simulink model "SF009A_DutyCycThermProtn"  (R2013b)
settings: Solver=FixedStepDiscrete  SolverMode=SingleTasking  StartTime=0.0  StopTime=1  FixedStep=0.1  RelTol=1e-3
values from neighbouring files (symbols this model uses):
  AbsltTThermLimCnt = DataDict.NTC    [SF009A_DutyCycThermProtn_DataDict.m]
  ARCHGLBPRM_100MILLISEC_SEC_F32 = DataDict.Constant    [SF009A_DutyCycThermProtn_DataDict.m]
  CTRLRANDCUTFLT_CNT_U08 = DataDict.Constant    [SF009A_DutyCycThermProtn_DataDict.m]
  CTRLRTFLT_CNT_U08 = DataDict.Constant    [SF009A_DutyCycThermProtn_DataDict.m]
  CUTFLT_CNT_U08 = DataDict.Constant    [SF009A_DutyCycThermProtn_DataDict.m]
  DITHERMLIM_MOTNWTMTR_F32 = DataDict.Constant    [SF009A_DutyCycThermProtn_DataDict.m]
  DutyCycExcddCnt = DataDict.NTC    [SF009A_DutyCycThermProtn_DataDict.m]
  DutyCycThermProtnAbsltCtrlTTblX = DataDict.Calibration    [SF009A_DutyCycThermProtn_DataDict.m]
  DutyCycThermProtnAbsltCtrlTTqTblY = DataDict.Calibration    [SF009A_DutyCycThermProtn_DataDict.m]
  DutyCycThermProtnAbsltCuTTblX = DataDict.Calibration    [SF009A_DutyCycThermProtn_DataDict.m]
  DutyCycThermProtnAbsltCuTTqTblY = DataDict.Calibration    [SF009A_DutyCycThermProtn_DataDict.m]
  DutyCycThermProtnAbsltMotVelBreakPt = DataDict.Calibration    [SF009A_DutyCycThermProtn_DataDict.m]
  DutyCycThermProtnAbsltTTqSlewHiLim = DataDict.Calibration    [SF009A_DutyCycThermProtn_DataDict.m]
  DutyCycThermProtnAbsltTTqSlewLoLim = DataDict.Calibration    [SF009A_DutyCycThermProtn_DataDict.m]
  DutyCycThermProtnCtrlT = DataDict.Calibration    [SF009A_DutyCycThermProtn_DataDict.m]
  DutyCycThermProtnCtrlTSeln = DataDict.Calibration    [SF009A_DutyCycThermProtn_DataDict.m]
  DutyCycThermProtnDutyCycFildThd = DataDict.Calibration    [SF009A_DutyCycThermProtn_DataDict.m]
  DutyCycThermProtnIgnOffCtrlEna = DataDict.Calibration    [SF009A_DutyCycThermProtn_DataDict.m]
  DutyCycThermProtnIgnOffMsgWaitTi = DataDict.Calibration    [SF009A_DutyCycThermProtn_DataDict.m]
  DutyCycThermProtnLstTblValNonStall = DataDict.Calibration    [SF009A_DutyCycThermProtn_DataDict.m]
  DutyCycThermProtnLstTblValStall = DataDict.Calibration    [SF009A_DutyCycThermProtn_DataDict.m]
  DutyCycThermProtnMotPrTSeln = DataDict.Calibration    [SF009A_DutyCycThermProtn_DataDict.m]
  DutyCycThermProtnMplr1NonStallTblY = DataDict.Calibration    [SF009A_DutyCycThermProtn_DataDict.m]
  DutyCycThermProtnMplr1StallTblY = DataDict.Calibration    [SF009A_DutyCycThermProtn_DataDict.m]
  DutyCycThermProtnMplr2NonStallTblY = DataDict.Calibration    [SF009A_DutyCycThermProtn_DataDict.m]
  DutyCycThermProtnMplr2StallTblY = DataDict.Calibration    [SF009A_DutyCycThermProtn_DataDict.m]
  DutyCycThermProtnMplr3NonStallTblY = DataDict.Calibration    [SF009A_DutyCycThermProtn_DataDict.m]
  DutyCycThermProtnMplr3StallTblY = DataDict.Calibration    [SF009A_DutyCycThermProtn_DataDict.m]
  DutyCycThermProtnMplr4NonStallTblY = DataDict.Calibration    [SF009A_DutyCycThermProtn_DataDict.m]
  DutyCycThermProtnMplr4StallTblY = DataDict.Calibration    [SF009A_DutyCycThermProtn_DataDict.m]
  DutyCycThermProtnMplr5NonStallTblY = DataDict.Calibration    [SF009A_DutyCycThermProtn_DataDict.m]
  DutyCycThermProtnMplr5StallTblY = DataDict.Calibration    [SF009A_DutyCycThermProtn_DataDict.m]
  DutyCycThermProtnMplr6NonStallTblY = DataDict.Calibration    [SF009A_DutyCycThermProtn_DataDict.m]
  DutyCycThermProtnMplr6StallTblY = DataDict.Calibration    [SF009A_DutyCycThermProtn_DataDict.m]
  DutyCycThermProtnMplrTblX = DataDict.Calibration    [SF009A_DutyCycThermProtn_DataDict.m]
  DutyCycThermProtnMplrTSeln = DataDict.Calibration    [SF009A_DutyCycThermProtn_DataDict.m]
  DutyCycThermProtnSlowFilTSeln = DataDict.Calibration    [SF009A_DutyCycThermProtn_DataDict.m]
  DutyCycThermProtnThermLimScaFac = DataDict.Calibration    [SF009A_DutyCycThermProtn_DataDict.m]
  DutyCycThermProtnThermLoadLimTblX = DataDict.Calibration    [SF009A_DutyCycThermProtn_DataDict.m]
  DutyCycThermProtnThermLoadLimTblY = DataDict.Calibration    [SF009A_DutyCycThermProtn_DataDict.m]
  DutyCycThermProtnTqCmdSlewDwn = DataDict.Calibration    [SF009A_DutyCycThermProtn_DataDict.m]
  DutyCycThermProtnTqCmdSlewUp = DataDict.Calibration    [SF009A_DutyCycThermProtn_DataDict.m]
  FILVALMIN_ULS_F32 = DataDict.Constant    [SF009A_DutyCycThermProtn_DataDict.m]
  IGNTIOFFTHD_CNT_F32 = DataDict.Constant    [SF009A_DutyCycThermProtn_DataDict.m]
  NODEBSTEP_CNT_U16 = DataDict.Constant    [SF009A_DutyCycThermProtn_DataDict.m]
  ONEPERC_ULS_F32 = DataDict.Constant    [SF009A_DutyCycThermProtn_DataDict.m]
  TAU3_SEC_F32 = DataDict.Constant    [SF009A_DutyCycThermProtn_DataDict.m]
  TAU4_SEC_F32 = DataDict.Constant    [SF009A_DutyCycThermProtn_DataDict.m]
  TAU5_SEC_F32 = DataDict.Constant    [SF009A_DutyCycThermProtn_DataDict.m]
  TAU6_SEC_F32 = DataDict.Constant    [SF009A_DutyCycThermProtn_DataDict.m]
  THERMLOADLIMTBLIDX_ULS_U08 = DataDict.Constant    [SF009A_DutyCycThermProtn_DataDict.m]
undefined symbols (not defined in the file or in its folder): NtcSts1, NvmGetErrSts1
libraries: FixdToFloat x13, Fil x12, NxtrLim x12, simulink x11, NxtrMath x8, FloatToFixd x6, NxtrMax x6, NxtrMin x3, NxtrAbslt x2, NxtrNvM x1
(part 5 of 7)

== system SF009A_DutyCycThermProtn/DutyCycThermProtn/DutyCycThermProtnPer1/TherrmalLimitScaling/ThermDutyCycLoadDptDisabled  ==
  Action Port : ActionPort  ActionType=then
  CopyRight2 : Subsystem  Description=|  mask(Copyright Information){none=on}
      | Copyright info block.                                               
      |                                                                     
      | Place copyright information at the top of every subsystem in design.
      mask prompts: none "No parameters"
      mask help: Place copyright information at the top of every subsystem in design.
      mask Display:
      | NxtrConf = 'Nexteer Confidential';
      | 
      | sys = bdroot; %handle for the current model ("system")
      | first = get_param(sys,'Created');
      | first = first(end-3:end);  %year is last four digits
      | 
      | last = get_param(sys,'LastModifiedDate');
      | if isempty(last)
      |     last = datestr(now,'yyyy');
      | else
      |     last = last(end-3:end);
      | end
      | 
      | if strcmp(first,last)
      |     fprintf('%s -- Copyright %s Nexteer',NxtrConf,first)
      | else
      |     fprintf('%s -- %s%s- %s Nexteer',NxtrConf,char(169),first,last)
      | end
  D_DEFEATTHERMLLIMIT_MTRNM : Constant  RequirementInfo="{'linktype_rmi_doors' '0000a52a (/E-STEER Core/SubSystem Specifications/Application Functions/SF009A Thermal Duty Cycle Protection)' '#SF009A_233' 'true' 'REQ:  SF009A_233' '' } %GIDa_fe9f7413_b640_416a_8163_cba554ef26c1"  Value=DITHERMLIM_MOTNWTMTR_F32
  ThermLdDptLim : Outport
  wires:
  D_DEFEATTHERMLLIMIT_MTRNM/1 -> ThermLdDptLim/1

== system SF009A_DutyCycThermProtn/DutyCycThermProtn/DutyCycThermProtnPer1/TherrmalLimitScaling/ThermDutyCycLoadDptEnabled ==
  ThermLoadDptLim : Inport
  Action Port : ActionPort  ActionType=else
  CopyRight2 : Subsystem  Description=|  mask(Copyright Information){none=on}
      | Copyright info block.                                               
      |                                                                     
      | Place copyright information at the top of every subsystem in design.
      mask prompts: none "No parameters"
      mask help: Place copyright information at the top of every subsystem in design.
      mask Display:
      | NxtrConf = 'Nexteer Confidential';
      | 
      | sys = bdroot; %handle for the current model ("system")
      | first = get_param(sys,'Created');
      | first = first(end-3:end);  %year is last four digits
      | 
      | last = get_param(sys,'LastModifiedDate');
      | if isempty(last)
      |     last = datestr(now,'yyyy');
      | else
      |     last = last(end-3:end);
      | end
      | 
      | if strcmp(first,last)
      |     fprintf('%s -- Copyright %s Nexteer',NxtrConf,first)
      | else
      |     fprintf('%s -- %s%s- %s Nexteer',NxtrConf,char(169),first,last)
      | end
  ThermLdDptLim : Outport
  wires:
  ThermLoadDptLim/1 -> ThermLdDptLim/1

== system SF009A_DutyCycThermProtn/DutyCycThermProtn/DutyCycThermProtnPer1/TherrmalLimitScaling/ThermLim_DutyCycThermProtnDisabled1 ==
  AbsTempLimitSlew : Inport
  Action Port : ActionPort  ActionType=then
  CopyRight2 : Subsystem  Description=|  mask(Copyright Information){none=on}
      | Copyright info block.                                               
      |                                                                     
      | Place copyright information at the top of every subsystem in design.
      mask prompts: none "No parameters"
      mask help: Place copyright information at the top of every subsystem in design.
      mask Display:
      | NxtrConf = 'Nexteer Confidential';
      | 
      | sys = bdroot; %handle for the current model ("system")
      | first = get_param(sys,'Created');
      | first = first(end-3:end);  %year is last four digits
      | 
      | last = get_param(sys,'LastModifiedDate');
      | if isempty(last)
      |     last = datestr(now,'yyyy');
      | else
      |     last = last(end-3:end);
      | end
      | 
      | if strcmp(first,last)
      |     fprintf('%s -- Copyright %s Nexteer',NxtrConf,first)
      | else
      |     fprintf('%s -- %s%s- %s Nexteer',NxtrConf,char(169),first,last)
      | end
  D_DEFEATTHERMLLIMIT_MTRNM : Constant  RequirementInfo="{'linktype_rmi_doors' '0000a52a (/E-STEER Core/SubSystem Specifications/Application Functions/SF009A Thermal Duty Cycle Protection)' '#SF009A_315' 'true' 'REQ:  SF009A_315' '' ; 'linktype_rmi_doors' '0000a52a (/E-STEER Core/SubSystem Specifications/Application Functions/SF009A Thermal Duty Cycle Protection)' '#SF009A_321' 'true' 'REQ:  SF009A_321' '' ; 'linktype_rmi_doors' '0000a52a (/E-STEER Core/SubSystem Specifications/Application Functions/SF009A Thermal Duty Cycle Protection)' '#SF009A_320' 'true' 'REQ:  SF009A_320' '' } %GIDa_b0686dc6_4c24_4aa9_95e9_6eecdcdad624"  Value=DutyCycThermProtnThermLimScaFac
  Product1 : Product  RndMeth=Zero
  ThermTempDptLmt : Outport
  wires:
  D_DEFEATTHERMLLIMIT_MTRNM/1 -> Product1/2
  Product1/1 -> ThermTempDptLmt/1
  AbsTempLimitSlew/1 -> Product1/1

== system SF009A_DutyCycThermProtn/DutyCycThermProtn/DutyCycThermProtnPer1/TherrmalLimitScaling/ThermLim_DutyCycThermProtnDisabled2 ==
  ThermalLoadLmt : Inport
  Action Port : ActionPort  ActionType=then
  CopyRight2 : Subsystem  Description=|  mask(Copyright Information){none=on}
      | Copyright info block.                                               
      |                                                                     
      | Place copyright information at the top of every subsystem in design.
      mask prompts: none "No parameters"
      mask help: Place copyright information at the top of every subsystem in design.
      mask Display:
      | NxtrConf = 'Nexteer Confidential';
      | 
      | sys = bdroot; %handle for the current model ("system")
      | first = get_param(sys,'Created');
      | first = first(end-3:end);  %year is last four digits
      | 
      | last = get_param(sys,'LastModifiedDate');
      | if isempty(last)
      |     last = datestr(now,'yyyy');
      | else
      |     last = last(end-3:end);
      | end
      | 
      | if strcmp(first,last)
      |     fprintf('%s -- Copyright %s Nexteer',NxtrConf,first)
      | else
      |     fprintf('%s -- %s%s- %s Nexteer',NxtrConf,char(169),first,last)
      | end
  D_DEFEATTHERMLLIMIT_MTRNM : Constant  RequirementInfo="{'linktype_rmi_doors' '0000a52a (/E-STEER Core/SubSystem Specifications/Application Functions/SF009A Thermal Duty Cycle Protection)' '#SF009A_315' 'true' 'REQ:  SF009A_315' '' ; 'linktype_rmi_doors' '0000a52a (/E-STEER Core/SubSystem Specifications/Application Functions/SF009A Thermal Duty Cycle Protection)' '#SF009A_320' 'true' 'REQ:  SF009A_320' '' ; 'linktype_rmi_doors' '0000a52a (/E-STEER Core/SubSystem Specifications/Application Functions/SF009A Thermal Duty Cycle Protection)' '#SF009A_321' 'true' 'REQ:  SF009A_321' '' } %GIDa_bbfb0ab5_887d_4318_9632_7a302babdc5f"  Value=DutyCycThermProtnThermLimScaFac
  Product1 : Product  RndMeth=Zero
  ThermLoadDptLim : Outport
  wires:
  D_DEFEATTHERMLLIMIT_MTRNM/1 -> Product1/2
  Product1/1 -> ThermLoadDptLim/1
  ThermalLoadLmt/1 -> Product1/1

== system SF009A_DutyCycThermProtn/DutyCycThermProtn/DutyCycThermProtnPer1/TherrmalLimitScaling/ThermLim_DutyCycThermProtnEnabled1 ==
  AbsTempLimitSlew : Inport
  Action Port : ActionPort  ActionType=else
  CopyRight2 : Subsystem  Description=|  mask(Copyright Information){none=on}
      | Copyright info block.                                               
      |                                                                     
      | Place copyright information at the top of every subsystem in design.
      mask prompts: none "No parameters"
      mask help: Place copyright information at the top of every subsystem in design.
      mask Display:
      | NxtrConf = 'Nexteer Confidential';
      | 
      | sys = bdroot; %handle for the current model ("system")
      | first = get_param(sys,'Created');
      | first = first(end-3:end);  %year is last four digits
      | 
      | last = get_param(sys,'LastModifiedDate');
      | if isempty(last)
      |     last = datestr(now,'yyyy');
      | else
      |     last = last(end-3:end);
      | end
      | 
      | if strcmp(first,last)
      |     fprintf('%s -- Copyright %s Nexteer',NxtrConf,first)
      | else
      |     fprintf('%s -- %s%s- %s Nexteer',NxtrConf,char(169),first,last)
      | end
  ThermTempDptLmt : Outport
  wires:
  AbsTempLimitSlew/1 -> ThermTempDptLmt/1

== system SF009A_DutyCycThermProtn/DutyCycThermProtn/DutyCycThermProtnPer1/TherrmalLimitScaling/ThermLim_DutyCycThermProtnEnabled2 ==
  ThermalLoadLmt : Inport
  Action Port : ActionPort  ActionType=else
  CopyRight2 : Subsystem  Description=|  mask(Copyright Information){none=on}
      | Copyright info block.                                               
      |                                                                     
      | Place copyright information at the top of every subsystem in design.
      mask prompts: none "No parameters"
      mask help: Place copyright information at the top of every subsystem in design.
      mask Display:
      | NxtrConf = 'Nexteer Confidential';
      | 
      | sys = bdroot; %handle for the current model ("system")
      | first = get_param(sys,'Created');
      | first = first(end-3:end);  %year is last four digits
      | 
      | last = get_param(sys,'LastModifiedDate');
      | if isempty(last)
      |     last = datestr(now,'yyyy');
      | else
      |     last = last(end-3:end);
      | end
      | 
      | if strcmp(first,last)
      |     fprintf('%s -- Copyright %s Nexteer',NxtrConf,first)
      | else
      |     fprintf('%s -- %s%s- %s Nexteer',NxtrConf,char(169),first,last)
      | end
  ThermLoadDptLim : Outport
  wires:
  ThermalLoadLmt/1 -> ThermLoadDptLim/1

== system SF009A_DutyCycThermProtn/DutyCycThermProtn/DutyCycThermProtnInit1/PowerOnTasks/DefaultIgnOffTime/CopyRight2 ==

== system SF009A_DutyCycThermProtn/DutyCycThermProtn/DutyCycThermProtnInit1/PowerOnTasks/InputIgnOffTime/CopyRight2 ==

== system SF009A_DutyCycThermProtn/DutyCycThermProtn/DutyCycThermProtnInit1/PowerOnTasks/InputIgnOffTime/Filt3ExpDecay ==
  IgnTimeOffSel : Inport  RequirementInfo={'linktype_rmi_doors' '0000a52a (/E-STEER Core/SubSystem Specifications/Application Functions/SF009A Thermal Duty Cycle Protection)' '#SF009A_285' 'true' 'REQ: SF009A_285' '' } %GIDa_5c5cb044_26c8_4dbf_bfdb_5ff65517aeea
  FiltSVOrg : Inport  RequirementInfo={'linktype_rmi_doors' '0000a52a (/E-STEER Core/SubSystem Specifications/Application Functions/SF009A Thermal Duty Cycle Protection)' '#SF009A_285' 'true' 'REQ: SF009A_285' '' } %GIDa_91a7a242_3564_4b75_930d_3be3ef1f28fd  Port=2
  CopyRight2 : Subsystem  Description=|  mask(Copyright Information){none=on}
      | Copyright info block.                                               
      |                                                                     
      | Place copyright information at the top of every subsystem in design.
      mask prompts: none "No parameters"
      mask help: Place copyright information at the top of every subsystem in design.
      mask Display:
      | NxtrConf = 'Nexteer Confidential';
      | 
      | sys = bdroot; %handle for the current model ("system")
      | first = get_param(sys,'Created');
      | first = first(end-3:end);  %year is last four digits
      | 
      | last = get_param(sys,'LastModifiedDate');
      | if isempty(last)
      |     last = datestr(now,'yyyy');
      | else
      |     last = last(end-3:end);
      | end
      | 
      | if strcmp(first,last)
      |     fprintf('%s -- Copyright %s Nexteer',NxtrConf,first)
      | else
      |     fprintf('%s -- %s%s- %s Nexteer',NxtrConf,char(169),first,last)
      | end
  Exp_f32 : NxtrMath/Exp_f32  RequirementInfo={'linktype_rmi_doors' '0000a52a (/E-STEER Core/SubSystem Specifications/Application Functions/SF009A Thermal Duty Cycle Protection)' '#SF009A_285' 'true' 'REQ: SF009A_285' '' } %GIDa_7883efea_e5ae_4044_b7ed_02762036b56f  SFunctionSpec=single y1 = Exp_f32(single u1)  ShowSpec=on
      settings: AttributesFormatString=%<MaskType>
  Gain : Gain  RequirementInfo={'linktype_rmi_doors' '0000a52a (/E-STEER Core/SubSystem Specifications/Application Functions/SF009A Thermal Duty Cycle Protection)' '#SF009A_285' 'true' 'REQ: SF009A_285' '' } %GIDa_88cc6e5b_9aec_42fe_9fe2_a5cfa1021eda  Gain=-1
  Product1 : Product  RequirementInfo={'linktype_rmi_doors' '0000a52a (/E-STEER Core/SubSystem Specifications/Application Functions/SF009A Thermal Duty Cycle Protection)' '#SF009A_285' 'true' 'REQ: SF009A_285' '' } %GIDa_0fcfcda3_a01a_4d7a_af05_1e45f2a4ef74  RndMeth=Zero
  Product2 : Product  RequirementInfo={'linktype_rmi_doors' '0000a52a (/E-STEER Core/SubSystem Specifications/Application Functions/SF009A Thermal Duty Cycle Protection)' '#SF009A_285' 'true' 'REQ: SF009A_285' '' } %GIDa_261a80b6_5869_428e_8277_22821d348308  Inputs=*/  RndMeth=Zero
  Tau : Constant  RequirementInfo={'linktype_rmi_doors' '0000a52a (/E-STEER Core/SubSystem Specifications/Application Functions/SF009A Thermal Duty Cycle Protection)' '#SF009A_285' 'true' 'REQ: SF009A_285' '' } %GIDa_03bc81ed_1d96_46ca_851c_5da21a8f4976  Value=TAU3_SEC_F32
  FiltSV : Outport  RequirementInfo={'linktype_rmi_doors' '0000a52a (/E-STEER Core/SubSystem Specifications/Application Functions/SF009A Thermal Duty Cycle Protection)' '#SF009A_285' 'true' 'REQ: SF009A_285' '' } %GIDa_bdc8e6b7_90e9_4d60_8279_bf082cc585c6
  wires:
  FiltSVOrg/1 -> Product1/2
  Product1/1 -> FiltSV/1
  IgnTimeOffSel/1 -> Gain/1
  Tau/1 -> Product2/2
  Exp_f32/1 -> Product1/1
  Gain/1 -> Product2/1
  Product2/1 -> Exp_f32/1

== system SF009A_DutyCycThermProtn/DutyCycThermProtn/DutyCycThermProtnInit1/PowerOnTasks/InputIgnOffTime/Filt4ExpDecay ==
  IgnTimeOffSel : Inport  RequirementInfo={'linktype_rmi_doors' '0000a52a (/E-STEER Core/SubSystem Specifications/Application Functions/SF009A Thermal Duty Cycle Protection)' '#SF009A_285' 'true' 'REQ: SF009A_285' '' } %GIDa_7550d9c9_f333_4982_a7f0_be5fb272d54b
  FiltSVOrg : Inport  RequirementInfo={'linktype_rmi_doors' '0000a52a (/E-STEER Core/SubSystem Specifications/Application Functions/SF009A Thermal Duty Cycle Protection)' '#SF009A_285' 'true' 'REQ: SF009A_285' '' } %GIDa_0ac67eff_405d_4d9d_b637_6c1188d91fb4  Port=2
  CopyRight2 : Subsystem  Description=|  mask(Copyright Information){none=on}
      | Copyright info block.                                               
      |                                                                     
      | Place copyright information at the top of every subsystem in design.
      mask prompts: none "No parameters"
      mask help: Place copyright information at the top of every subsystem in design.
      mask Display:
      | NxtrConf = 'Nexteer Confidential';
      | 
      | sys = bdroot; %handle for the current model ("system")
      | first = get_param(sys,'Created');
      | first = first(end-3:end);  %year is last four digits
      | 
      | last = get_param(sys,'LastModifiedDate');
      | if isempty(last)
      |     last = datestr(now,'yyyy');
      | else
      |     last = last(end-3:end);
      | end
      | 
      | if strcmp(first,last)
      |     fprintf('%s -- Copyright %s Nexteer',NxtrConf,first)
      | else
      |     fprintf('%s -- %s%s- %s Nexteer',NxtrConf,char(169),first,last)
      | end
  Exp_f32 : NxtrMath/Exp_f32  RequirementInfo={'linktype_rmi_doors' '0000a52a (/E-STEER Core/SubSystem Specifications/Application Functions/SF009A Thermal Duty Cycle Protection)' '#SF009A_285' 'true' 'REQ: SF009A_285' '' } %GIDa_57703fab_89c6_46b9_a010_6a300dd59952  SFunctionSpec=single y1 = Exp_f32(single u1)  ShowSpec=on
      settings: AttributesFormatString=%<MaskType>
  Gain : Gain  RequirementInfo={'linktype_rmi_doors' '0000a52a (/E-STEER Core/SubSystem Specifications/Application Functions/SF009A Thermal Duty Cycle Protection)' '#SF009A_285' 'true' 'REQ: SF009A_285' '' } %GIDa_c87ee9d0_4095_4a61_9d3d_879e8b6486a8  Gain=-1
  Product1 : Product  RequirementInfo={'linktype_rmi_doors' '0000a52a (/E-STEER Core/SubSystem Specifications/Application Functions/SF009A Thermal Duty Cycle Protection)' '#SF009A_285' 'true' 'REQ: SF009A_285' '' } %GIDa_57d5ea56_1e55_4e31_b3e0_93aa11516aa8  RndMeth=Zero
  Product2 : Product  RequirementInfo={'linktype_rmi_doors' '0000a52a (/E-STEER Core/SubSystem Specifications/Application Functions/SF009A Thermal Duty Cycle Protection)' '#SF009A_285' 'true' 'REQ: SF009A_285' '' } %GIDa_750dcb34_2abd_4894_bf5e_3b0e89131671  Inputs=*/  RndMeth=Zero
  Tau : Constant  RequirementInfo={'linktype_rmi_doors' '0000a52a (/E-STEER Core/SubSystem Specifications/Application Functions/SF009A Thermal Duty Cycle Protection)' '#SF009A_285' 'true' 'REQ: SF009A_285' '' } %GIDa_b90e2574_3590_40ba_956f_a384e0479c3c  Value=TAU4_SEC_F32
  FiltSV : Outport  RequirementInfo={'linktype_rmi_doors' '0000a52a (/E-STEER Core/SubSystem Specifications/Application Functions/SF009A Thermal Duty Cycle Protection)' '#SF009A_285' 'true' 'REQ: SF009A_285' '' } %GIDa_35520a0b_7ea8_496f_ac90_73364029aadc
  wires:
  FiltSVOrg/1 -> Product1/2
  Product1/1 -> FiltSV/1
  IgnTimeOffSel/1 -> Gain/1
  Tau/1 -> Product2/2
  Exp_f32/1 -> Product1/1
  Product2/1 -> Exp_f32/1
  Gain/1 -> Product2/1

== system SF009A_DutyCycThermProtn/DutyCycThermProtn/DutyCycThermProtnInit1/PowerOnTasks/InputIgnOffTime/Filt5ExpDecay ==
  IgnTimeOffSel : Inport  RequirementInfo={'linktype_rmi_doors' '0000a52a (/E-STEER Core/SubSystem Specifications/Application Functions/SF009A Thermal Duty Cycle Protection)' '#SF009A_285' 'true' 'REQ: SF009A_285' '' } %GIDa_b90161fb_4064_45d7_9d6b_cab682484744
  FiltSVOrg : Inport  RequirementInfo={'linktype_rmi_doors' '0000a52a (/E-STEER Core/SubSystem Specifications/Application Functions/SF009A Thermal Duty Cycle Protection)' '#SF009A_285' 'true' 'REQ: SF009A_285' '' } %GIDa_f17c0eee_319f_4b2a_a1b3_070a9180d2cb  Port=2
  CopyRight2 : Subsystem  Description=|  mask(Copyright Information){none=on}
      | Copyright info block.                                               
      |                                                                     
      | Place copyright information at the top of every subsystem in design.
      mask prompts: none "No parameters"
      mask help: Place copyright information at the top of every subsystem in design.
      mask Display:
      | NxtrConf = 'Nexteer Confidential';
      | 
      | sys = bdroot; %handle for the current model ("system")
      | first = get_param(sys,'Created');
      | first = first(end-3:end);  %year is last four digits
      | 
      | last = get_param(sys,'LastModifiedDate');
      | if isempty(last)
      |     last = datestr(now,'yyyy');
      | else
      |     last = last(end-3:end);
      | end
      | 
      | if strcmp(first,last)
      |     fprintf('%s -- Copyright %s Nexteer',NxtrConf,first)
      | else
      |     fprintf('%s -- %s%s- %s Nexteer',NxtrConf,char(169),first,last)
      | end
  Exp_f32 : NxtrMath/Exp_f32  RequirementInfo={'linktype_rmi_doors' '0000a52a (/E-STEER Core/SubSystem Specifications/Application Functions/SF009A Thermal Duty Cycle Protection)' '#SF009A_285' 'true' 'REQ: SF009A_285' '' } %GIDa_aca0274c_5d2f_4959_ab19_73663ecd45f4  SFunctionSpec=single y1 = Exp_f32(single u1)  ShowSpec=on
      settings: AttributesFormatString=%<MaskType>
  Gain : Gain  RequirementInfo={'linktype_rmi_doors' '0000a52a (/E-STEER Core/SubSystem Specifications/Application Functions/SF009A Thermal Duty Cycle Protection)' '#SF009A_285' 'true' 'REQ: SF009A_285' '' } %GIDa_4e414b39_97a9_4e9b_aa01_66e532f180aa  Gain=-1
  Product1 : Product  RequirementInfo={'linktype_rmi_doors' '0000a52a (/E-STEER Core/SubSystem Specifications/Application Functions/SF009A Thermal Duty Cycle Protection)' '#SF009A_285' 'true' 'REQ: SF009A_285' '' } %GIDa_3ff6f461_99a4_4da1_aecf_e72e027f0494  RndMeth=Zero
  Product2 : Product  RequirementInfo={'linktype_rmi_doors' '0000a52a (/E-STEER Core/SubSystem Specifications/Application Functions/SF009A Thermal Duty Cycle Protection)' '#SF009A_285' 'true' 'REQ: SF009A_285' '' } %GIDa_a1ba9507_d090_4b6b_9d20_3c1727d1ce95  Inputs=*/  RndMeth=Zero
  Tau : Constant  RequirementInfo={'linktype_rmi_doors' '0000a52a (/E-STEER Core/SubSystem Specifications/Application Functions/SF009A Thermal Duty Cycle Protection)' '#SF009A_285' 'true' 'REQ: SF009A_285' '' } %GIDa_3c638df1_c7fd_4e50_a802_ff31d0fe74ad  Value=TAU5_SEC_F32
  FiltSV : Outport  RequirementInfo={'linktype_rmi_doors' '0000a52a (/E-STEER Core/SubSystem Specifications/Application Functions/SF009A Thermal Duty Cycle Protection)' '#SF009A_285' 'true' 'REQ: SF009A_285' '' } %GIDa_34068f8f_8835_45d5_8e2c_de5fc32af880
  wires:
  FiltSVOrg/1 -> Product1/2
  Product1/1 -> FiltSV/1
  IgnTimeOffSel/1 -> Gain/1
  Tau/1 -> Product2/2
  Exp_f32/1 -> Product1/1
  Product2/1 -> Exp_f32/1
  Gain/1 -> Product2/1

== system SF009A_DutyCycThermProtn/DutyCycThermProtn/DutyCycThermProtnInit1/PowerOnTasks/InputIgnOffTime/Filt6ExpDecay ==
  IgnTimeOffSel : Inport  RequirementInfo={'linktype_rmi_doors' '0000a52a (/E-STEER Core/SubSystem Specifications/Application Functions/SF009A Thermal Duty Cycle Protection)' '#SF009A_285' 'true' 'REQ: SF009A_285' '' } %GIDa_fdad97c5_2a7e_4b19_aee1_16e53b4fa469
  FiltSVOrg : Inport  RequirementInfo={'linktype_rmi_doors' '0000a52a (/E-STEER Core/SubSystem Specifications/Application Functions/SF009A Thermal Duty Cycle Protection)' '#SF009A_285' 'true' 'REQ: SF009A_285' '' } %GIDa_62f56edd_175f_4c7b_815e_c7943bed403b  Port=2
  CopyRight2 : Subsystem  Description=|  mask(Copyright Information){none=on}
      | Copyright info block.                                               
      |                                                                     
      | Place copyright information at the top of every subsystem in design.
      mask prompts: none "No parameters"
      mask help: Place copyright information at the top of every subsystem in design.
      mask Display:
      | NxtrConf = 'Nexteer Confidential';
      | 
      | sys = bdroot; %handle for the current model ("system")
      | first = get_param(sys,'Created');
      | first = first(end-3:end);  %year is last four digits
      | 
      | last = get_param(sys,'LastModifiedDate');
      | if isempty(last)
      |     last = datestr(now,'yyyy');
      | else
      |     last = last(end-3:end);
      | end
      | 
      | if strcmp(first,last)
      |     fprintf('%s -- Copyright %s Nexteer',NxtrConf,first)
      | else
      |     fprintf('%s -- %s%s- %s Nexteer',NxtrConf,char(169),first,last)
      | end
  Exp_f32 : NxtrMath/Exp_f32  RequirementInfo={'linktype_rmi_doors' '0000a52a (/E-STEER Core/SubSystem Specifications/Application Functions/SF009A Thermal Duty Cycle Protection)' '#SF009A_285' 'true' 'REQ: SF009A_285' '' } %GIDa_442b610e_7bae_4f5d_a580_07fd6a86bb9f  SFunctionSpec=single y1 = Exp_f32(single u1)  ShowSpec=on
      settings: AttributesFormatString=%<MaskType>
  Gain : Gain  RequirementInfo={'linktype_rmi_doors' '0000a52a (/E-STEER Core/SubSystem Specifications/Application Functions/SF009A Thermal Duty Cycle Protection)' '#SF009A_285' 'true' 'REQ: SF009A_285' '' } %GIDa_b39b7229_baa0_4654_9a01_936ece545f12  Gain=-1
  Product1 : Product  RequirementInfo={'linktype_rmi_doors' '0000a52a (/E-STEER Core/SubSystem Specifications/Application Functions/SF009A Thermal Duty Cycle Protection)' '#SF009A_285' 'true' 'REQ: SF009A_285' '' } %GIDa_63ecbc7b_6765_47a2_aab0_c4aabe4b6ba4  RndMeth=Zero
  Product2 : Product  RequirementInfo={'linktype_rmi_doors' '0000a52a (/E-STEER Core/SubSystem Specifications/Application Functions/SF009A Thermal Duty Cycle Protection)' '#SF009A_285' 'true' 'REQ: SF009A_285' '' } %GIDa_7bd2ccc2_3f25_47c1_a9ea_e44af7634a29  Inputs=*/  RndMeth=Zero
  Tau : Constant  RequirementInfo={'linktype_rmi_doors' '0000a52a (/E-STEER Core/SubSystem Specifications/Application Functions/SF009A Thermal Duty Cycle Protection)' '#SF009A_285' 'true' 'REQ: SF009A_285' '' } %GIDa_9b08b9e4_ef81_4b23_b03d_82f472a8b4ee  Value=TAU6_SEC_F32
  FiltSV : Outport  RequirementInfo={'linktype_rmi_doors' '0000a52a (/E-STEER Core/SubSystem Specifications/Application Functions/SF009A Thermal Duty Cycle Protection)' '#SF009A_285' 'true' 'REQ: SF009A_285' '' } %GIDa_7a9019c6_2f75_4e61_ae74_87f156da8ec8
  wires:
  FiltSVOrg/1 -> Product1/2
  Product1/1 -> FiltSV/1
  IgnTimeOffSel/1 -> Gain/1
  Tau/1 -> Product2/2
  Exp_f32/1 -> Product1/1
  Product2/1 -> Exp_f32/1
  Gain/1 -> Product2/1

== system SF009A_DutyCycThermProtn/DutyCycThermProtn/DutyCycThermProtnPer1/FiltSVReinit/VehTiVldDisabled/CopyRight2 ==

== system SF009A_DutyCycThermProtn/DutyCycThermProtn/DutyCycThermProtnPer1/FiltSVReinit/VehTiVldEnabled/CopyRight2 ==

== system SF009A_DutyCycThermProtn/DutyCycThermProtn/DutyCycThermProtnPer1/FiltSVReinit/VehTiVldEnabled/Filt3ExpDecay ==
  IgnTimeOffSel : Inport  RequirementInfo={'linktype_rmi_doors' '0000a52a (/E-STEER Core/SubSystem Specifications/Application Functions/SF009A Thermal Duty Cycle Protection)' '#SF009A_285' 'true' 'REQ: SF009A_285' '' } %GIDa_2f277cfa_04f7_4efd_8183_f26cc3ec11e8
  FiltSVOrg : Inport  RequirementInfo={'linktype_rmi_doors' '0000a52a (/E-STEER Core/SubSystem Specifications/Application Functions/SF009A Thermal Duty Cycle Protection)' '#SF009A_285' 'true' 'REQ: SF009A_285' '' } %GIDa_6a80f34d_15bd_486f_9b83_6a28aa3fe0ad  Port=2
  CopyRight2 : Subsystem  Description=|  mask(Copyright Information){none=on}
      | Copyright info block.                                               
      |                                                                     
      | Place copyright information at the top of every subsystem in design.
      mask prompts: none "No parameters"
      mask help: Place copyright information at the top of every subsystem in design.
      mask Display:
      | NxtrConf = 'Nexteer Confidential';
      | 
      | sys = bdroot; %handle for the current model ("system")
      | first = get_param(sys,'Created');
      | first = first(end-3:end);  %year is last four digits
      | 
      | last = get_param(sys,'LastModifiedDate');
      | if isempty(last)
      |     last = datestr(now,'yyyy');
      | else
      |     last = last(end-3:end);
      | end
      | 
      | if strcmp(first,last)
      |     fprintf('%s -- Copyright %s Nexteer',NxtrConf,first)
      | else
      |     fprintf('%s -- %s%s- %s Nexteer',NxtrConf,char(169),first,last)
      | end
  Exp_f32 : NxtrMath/Exp_f32  RequirementInfo={'linktype_rmi_doors' '0000a52a (/E-STEER Core/SubSystem Specifications/Application Functions/SF009A Thermal Duty Cycle Protection)' '#SF009A_285' 'true' 'REQ: SF009A_285' '' } %GIDa_b4229f1b_62cf_4fab_b7ac_5aae12ad4bab  SFunctionSpec=single y1 = Exp_f32(single u1)  ShowSpec=on
      settings: AttributesFormatString=%<MaskType>
  Gain : Gain  RequirementInfo={'linktype_rmi_doors' '0000a52a (/E-STEER Core/SubSystem Specifications/Application Functions/SF009A Thermal Duty Cycle Protection)' '#SF009A_285' 'true' 'REQ: SF009A_285' '' } %GIDa_812109e6_0a0a_42eb_b926_01a1c9078124  Gain=-1
  Product1 : Product  RequirementInfo={'linktype_rmi_doors' '0000a52a (/E-STEER Core/SubSystem Specifications/Application Functions/SF009A Thermal Duty Cycle Protection)' '#SF009A_285' 'true' 'REQ: SF009A_285' '' } %GIDa_513c209d_51b2_4ef5_92ed_fc68d3c652a9  RndMeth=Zero
  Product2 : Product  RequirementInfo={'linktype_rmi_doors' '0000a52a (/E-STEER Core/SubSystem Specifications/Application Functions/SF009A Thermal Duty Cycle Protection)' '#SF009A_285' 'true' 'REQ: SF009A_285' '' } %GIDa_9ed37af2_4fbf_4a4c_9446_92cf6ee91099  Inputs=*/  RndMeth=Zero
  Tau : Constant  RequirementInfo={'linktype_rmi_doors' '0000a52a (/E-STEER Core/SubSystem Specifications/Application Functions/SF009A Thermal Duty Cycle Protection)' '#SF009A_285' 'true' 'REQ: SF009A_285' '' } %GIDa_3ad883e5_7e2a_4b45_9df7_35a559f2c6ef  Value=TAU3_SEC_F32
  FiltSV : Outport  RequirementInfo={'linktype_rmi_doors' '0000a52a (/E-STEER Core/SubSystem Specifications/Application Functions/SF009A Thermal Duty Cycle Protection)' '#SF009A_285' 'true' 'REQ: SF009A_285' '' } %GIDa_d206a6cd_498c_40ce_9958_2f76665f34bf
  wires:
  FiltSVOrg/1 -> Product1/2
  Product1/1 -> FiltSV/1
  IgnTimeOffSel/1 -> Gain/1
  Tau/1 -> Product2/2
  Exp_f32/1 -> Product1/1
  Product2/1 -> Exp_f32/1
  Gain/1 -> Product2/1

== system SF009A_DutyCycThermProtn/DutyCycThermProtn/DutyCycThermProtnPer1/FiltSVReinit/VehTiVldEnabled/Filt4ExpDecay ==
  IgnTimeOffSel : Inport  RequirementInfo={'linktype_rmi_doors' '0000a52a (/E-STEER Core/SubSystem Specifications/Application Functions/SF009A Thermal Duty Cycle Protection)' '#SF009A_285' 'true' 'REQ: SF009A_285' '' } %GIDa_688e095e_1630_4ee3_972a_0461832cdda3
  FiltSVOrg : Inport  RequirementInfo={'linktype_rmi_doors' '0000a52a (/E-STEER Core/SubSystem Specifications/Application Functions/SF009A Thermal Duty Cycle Protection)' '#SF009A_285' 'true' 'REQ: SF009A_285' '' } %GIDa_33abdde2_151f_4fc4_9a55_e2f8223019fd  Port=2
  CopyRight2 : Subsystem  Description=|  mask(Copyright Information){none=on}
      | Copyright info block.                                               
      |                                                                     
      | Place copyright information at the top of every subsystem in design.
      mask prompts: none "No parameters"
      mask help: Place copyright information at the top of every subsystem in design.
      mask Display:
      | NxtrConf = 'Nexteer Confidential';
      | 
      | sys = bdroot; %handle for the current model ("system")
      | first = get_param(sys,'Created');
      | first = first(end-3:end);  %year is last four digits
      | 
      | last = get_param(sys,'LastModifiedDate');
      | if isempty(last)
      |     last = datestr(now,'yyyy');
      | else
      |     last = last(end-3:end);
      | end
      | 
      | if strcmp(first,last)
      |     fprintf('%s -- Copyright %s Nexteer',NxtrConf,first)
      | else
      |     fprintf('%s -- %s%s- %s Nexteer',NxtrConf,char(169),first,last)
      | end
  Exp_f32 : NxtrMath/Exp_f32  RequirementInfo={'linktype_rmi_doors' '0000a52a (/E-STEER Core/SubSystem Specifications/Application Functions/SF009A Thermal Duty Cycle Protection)' '#SF009A_285' 'true' 'REQ: SF009A_285' '' } %GIDa_9ab4e45b_1b1b_40ca_9537_5302fb2ce499  SFunctionSpec=single y1 = Exp_f32(single u1)  ShowSpec=on
      settings: AttributesFormatString=%<MaskType>
  Gain : Gain  RequirementInfo={'linktype_rmi_doors' '0000a52a (/E-STEER Core/SubSystem Specifications/Application Functions/SF009A Thermal Duty Cycle Protection)' '#SF009A_285' 'true' 'REQ: SF009A_285' '' } %GIDa_ae4547df_6077_493c_bd57_9f901f4fd88e  Gain=-1
  Product1 : Product  RequirementInfo={'linktype_rmi_doors' '0000a52a (/E-STEER Core/SubSystem Specifications/Application Functions/SF009A Thermal Duty Cycle Protection)' '#SF009A_285' 'true' 'REQ: SF009A_285' '' } %GIDa_0394ebf4_f70b_4d0f_9f33_5e25d2d33165  RndMeth=Zero
  Product2 : Product  RequirementInfo={'linktype_rmi_doors' '0000a52a (/E-STEER Core/SubSystem Specifications/Application Functions/SF009A Thermal Duty Cycle Protection)' '#SF009A_285' 'true' 'REQ: SF009A_285' '' } %GIDa_031938eb_88a5_4562_96f1_5b0d01f7e7d0  Inputs=*/  RndMeth=Zero
  Tau : Constant  RequirementInfo={'linktype_rmi_doors' '0000a52a (/E-STEER Core/SubSystem Specifications/Application Functions/SF009A Thermal Duty Cycle Protection)' '#SF009A_285' 'true' 'REQ: SF009A_285' '' } %GIDa_2afa65fd_4a07_43e0_808b_6dfeb622c5cf  Value=TAU4_SEC_F32
  FiltSV : Outport  RequirementInfo={'linktype_rmi_doors' '0000a52a (/E-STEER Core/SubSystem Specifications/Application Functions/SF009A Thermal Duty Cycle Protection)' '#SF009A_285' 'true' 'REQ: SF009A_285' '' } %GIDa_09e81401_3187_40f5_b989_31a238aef27e
  wires:
  FiltSVOrg/1 -> Product1/2
  Product1/1 -> FiltSV/1
  IgnTimeOffSel/1 -> Gain/1
  Tau/1 -> Product2/2
  Exp_f32/1 -> Product1/1
  Product2/1 -> Exp_f32/1
  Gain/1 -> Product2/1

== system SF009A_DutyCycThermProtn/DutyCycThermProtn/DutyCycThermProtnPer1/FiltSVReinit/VehTiVldEnabled/Filt5ExpDecay ==
  IgnTimeOffSel : Inport  RequirementInfo={'linktype_rmi_doors' '0000a52a (/E-STEER Core/SubSystem Specifications/Application Functions/SF009A Thermal Duty Cycle Protection)' '#SF009A_285' 'true' 'REQ: SF009A_285' '' } %GIDa_4b3c6625_036b_454a_a724_14ca2dcbb2da
  FiltSVOrg : Inport  RequirementInfo={'linktype_rmi_doors' '0000a52a (/E-STEER Core/SubSystem Specifications/Application Functions/SF009A Thermal Duty Cycle Protection)' '#SF009A_285' 'true' 'REQ: SF009A_285' '' } %GIDa_6a4306e6_23dd_484c_b80e_68c6e3bc06b4  Port=2
  CopyRight2 : Subsystem  Description=|  mask(Copyright Information){none=on}
      | Copyright info block.                                               
      |                                                                     
      | Place copyright information at the top of every subsystem in design.
      mask prompts: none "No parameters"
      mask help: Place copyright information at the top of every subsystem in design.
      mask Display:
      | NxtrConf = 'Nexteer Confidential';
      | 
      | sys = bdroot; %handle for the current model ("system")
      | first = get_param(sys,'Created');
      | first = first(end-3:end);  %year is last four digits
      | 
      | last = get_param(sys,'LastModifiedDate');
      | if isempty(last)
      |     last = datestr(now,'yyyy');
      | else
      |     last = last(end-3:end);
      | end
      | 
      | if strcmp(first,last)
      |     fprintf('%s -- Copyright %s Nexteer',NxtrConf,first)
      | else
      |     fprintf('%s -- %s%s- %s Nexteer',NxtrConf,char(169),first,last)
      | end
  Exp_f32 : NxtrMath/Exp_f32  RequirementInfo={'linktype_rmi_doors' '0000a52a (/E-STEER Core/SubSystem Specifications/Application Functions/SF009A Thermal Duty Cycle Protection)' '#SF009A_285' 'true' 'REQ: SF009A_285' '' } %GIDa_729f0013_7065_409d_b238_6136c9e3c98a  SFunctionSpec=single y1 = Exp_f32(single u1)  ShowSpec=on
      settings: AttributesFormatString=%<MaskType>
  Gain : Gain  RequirementInfo={'linktype_rmi_doors' '0000a52a (/E-STEER Core/SubSystem Specifications/Application Functions/SF009A Thermal Duty Cycle Protection)' '#SF009A_285' 'true' 'REQ: SF009A_285' '' } %GIDa_bbcc1544_a7e8_4ae1_a20b_cd0ae4505034  Gain=-1
  Product1 : Product  RequirementInfo={'linktype_rmi_doors' '0000a52a (/E-STEER Core/SubSystem Specifications/Application Functions/SF009A Thermal Duty Cycle Protection)' '#SF009A_285' 'true' 'REQ: SF009A_285' '' } %GIDa_be0cdc15_84dd_4bed_943b_4c704b26c2bc  RndMeth=Zero
  Product2 : Product  RequirementInfo={'linktype_rmi_doors' '0000a52a (/E-STEER Core/SubSystem Specifications/Application Functions/SF009A Thermal Duty Cycle Protection)' '#SF009A_285' 'true' 'REQ: SF009A_285' '' } %GIDa_314f3b14_1b37_4b85_9ca8_b369e9216989  Inputs=*/  RndMeth=Zero
  Tau : Constant  RequirementInfo={'linktype_rmi_doors' '0000a52a (/E-STEER Core/SubSystem Specifications/Application Functions/SF009A Thermal Duty Cycle Protection)' '#SF009A_285' 'true' 'REQ: SF009A_285' '' } %GIDa_d1fd6718_b6b6_439a_9b30_27e3c174fb58  Value=TAU5_SEC_F32
  FiltSV : Outport  RequirementInfo={'linktype_rmi_doors' '0000a52a (/E-STEER Core/SubSystem Specifications/Application Functions/SF009A Thermal Duty Cycle Protection)' '#SF009A_285' 'true' 'REQ: SF009A_285' '' } %GIDa_b586d7b9_90b1_4c51_9dde_316f6a7aeae4
  wires:
  FiltSVOrg/1 -> Product1/2
  Product1/1 -> FiltSV/1
  IgnTimeOffSel/1 -> Gain/1
  Tau/1 -> Product2/2
  Exp_f32/1 -> Product1/1
  Product2/1 -> Exp_f32/1
  Gain/1 -> Product2/1

== system SF009A_DutyCycThermProtn/DutyCycThermProtn/DutyCycThermProtnPer1/FiltSVReinit/VehTiVldEnabled/Filt6ExpDecay ==
  IgnTimeOffSel : Inport  RequirementInfo={'linktype_rmi_doors' '0000a52a (/E-STEER Core/SubSystem Specifications/Application Functions/SF009A Thermal Duty Cycle Protection)' '#SF009A_285' 'true' 'REQ: SF009A_285' '' } %GIDa_f5a9550d_806c_414d_8631_2d2380b76ab0
  FiltSVOrg : Inport  RequirementInfo={'linktype_rmi_doors' '0000a52a (/E-STEER Core/SubSystem Specifications/Application Functions/SF009A Thermal Duty Cycle Protection)' '#SF009A_285' 'true' 'REQ: SF009A_285' '' } %GIDa_2defac87_6e02_413b_8475_9d4c2cb69c9e  Port=2
  CopyRight2 : Subsystem  Description=|  mask(Copyright Information){none=on}
      | Copyright info block.                                               
      |                                                                     
      | Place copyright information at the top of every subsystem in design.
      mask prompts: none "No parameters"
      mask help: Place copyright information at the top of every subsystem in design.
      mask Display:
      | NxtrConf = 'Nexteer Confidential';
      | 
      | sys = bdroot; %handle for the current model ("system")
      | first = get_param(sys,'Created');
      | first = first(end-3:end);  %year is last four digits
      | 
      | last = get_param(sys,'LastModifiedDate');
      | if isempty(last)
      |     last = datestr(now,'yyyy');
      | else
      |     last = last(end-3:end);
      | end
      | 
      | if strcmp(first,last)
      |     fprintf('%s -- Copyright %s Nexteer',NxtrConf,first)
      | else
      |     fprintf('%s -- %s%s- %s Nexteer',NxtrConf,char(169),first,last)
      | end
  Exp_f32 : NxtrMath/Exp_f32  RequirementInfo={'linktype_rmi_doors' '0000a52a (/E-STEER Core/SubSystem Specifications/Application Functions/SF009A Thermal Duty Cycle Protection)' '#SF009A_285' 'true' 'REQ: SF009A_285' '' } %GIDa_4cd32e56_30f1_406e_b606_df838072ffb0  SFunctionSpec=single y1 = Exp_f32(single u1)  ShowSpec=on
      settings: AttributesFormatString=%<MaskType>
  Gain : Gain  RequirementInfo={'linktype_rmi_doors' '0000a52a (/E-STEER Core/SubSystem Specifications/Application Functions/SF009A Thermal Duty Cycle Protection)' '#SF009A_285' 'true' 'REQ: SF009A_285' '' } %GIDa_db36424d_59ba_47c6_b149_da317fa6ea06  Gain=-1
  Product1 : Product  RequirementInfo={'linktype_rmi_doors' '0000a52a (/E-STEER Core/SubSystem Specifications/Application Functions/SF009A Thermal Duty Cycle Protection)' '#SF009A_285' 'true' 'REQ: SF009A_285' '' } %GIDa_ddc8ce97_ddcc_41f8_8d8e_ba5cfb6ec71d  RndMeth=Zero
  Product2 : Product  RequirementInfo={'linktype_rmi_doors' '0000a52a (/E-STEER Core/SubSystem Specifications/Application Functions/SF009A Thermal Duty Cycle Protection)' '#SF009A_285' 'true' 'REQ: SF009A_285' '' } %GIDa_ce23dae0_90a7_4b7e_89df_c3a4364a01fe  Inputs=*/  RndMeth=Zero
  Tau : Constant  RequirementInfo={'linktype_rmi_doors' '0000a52a (/E-STEER Core/SubSystem Specifications/Application Functions/SF009A Thermal Duty Cycle Protection)' '#SF009A_285' 'true' 'REQ: SF009A_285' '' } %GIDa_9d922443_dae8_45b9_b8b2_6f88fda7eef6  Value=TAU6_SEC_F32
  FiltSV : Outport  RequirementInfo={'linktype_rmi_doors' '0000a52a (/E-STEER Core/SubSystem Specifications/Application Functions/SF009A Thermal Duty Cycle Protection)' '#SF009A_285' 'true' 'REQ: SF009A_285' '' } %GIDa_e2442da6_9164_440b_b69a_c1998b02fa69
  wires:
  FiltSVOrg/1 -> Product1/2
  Product1/1 -> FiltSV/1
  IgnTimeOffSel/1 -> Gain/1
  Tau/1 -> Product2/2
  Exp_f32/1 -> Product1/1
  Product2/1 -> Exp_f32/1
  Gain/1 -> Product2/1

== system SF009A_DutyCycThermProtn/DutyCycThermProtn/DutyCycThermProtnPer1/LoadLimiting/FilterPercMax/CopyRight2 ==

== system SF009A_DutyCycThermProtn/DutyCycThermProtn/DutyCycThermProtnPer1/LoadLimiting/FilterPercMax/DutyCycLevel_DutyCycThermProtnDisabled ==
  Action Port : ActionPort  ActionType=then
  CopyRight2 : Subsystem  Description=|  mask(Copyright Information){none=on}
      | Copyright info block.                                               
      |                                                                     
      | Place copyright information at the top of every subsystem in design.
      mask prompts: none "No parameters"
      mask help: Place copyright information at the top of every subsystem in design.
      mask Display:
      | NxtrConf = 'Nexteer Confidential';
      | 
      | sys = bdroot; %handle for the current model ("system")
      | first = get_param(sys,'Created');
      | first = first(end-3:end);  %year is last four digits
      | 
      | last = get_param(sys,'LastModifiedDate');
      | if isempty(last)
      |     last = datestr(now,'yyyy');
      | else
      |     last = last(end-3:end);
      | end
      | 
      | if strcmp(first,last)
      |     fprintf('%s -- Copyright %s Nexteer',NxtrConf,first)
      | else
      |     fprintf('%s -- %s%s- %s Nexteer',NxtrConf,char(169),first,last)
      | end
  D_DEFEATDUTYCYCLELEVEL_ULS : Constant  RequirementInfo={'linktype_rmi_doors' '0000a52a (/E-STEER Core/SubSystem Specifications/Application Functions/SF009A Thermal Duty Cycle Protection)' '#SF009A_168' 'true' 'REQ: SF009A_168' '' } %GIDa_cf1cd60c_14ff_436d_a874_5ee49fc952e4  Value=0  OutDataTypeStr=Inherit: Inherit via back propagation
  DutyCycleLevel : Outport
  wires:
  D_DEFEATDUTYCYCLELEVEL_ULS/1 -> DutyCycleLevel/1

== system SF009A_DutyCycThermProtn/DutyCycThermProtn/DutyCycThermProtnPer1/LoadLimiting/FilterPercMax/DutyCycLevel_DutyCycThermProtnEnabled ==
  MaxSlowFilt : Inport
  Action Port : ActionPort  ActionType=else
  CopyRight2 : Subsystem  Description=|  mask(Copyright Information){none=on}
      | Copyright info block.                                               
      |                                                                     
      | Place copyright information at the top of every subsystem in design.
      mask prompts: none "No parameters"
      mask help: Place copyright information at the top of every subsystem in design.
      mask Display:
      | NxtrConf = 'Nexteer Confidential';
      | 
      | sys = bdroot; %handle for the current model ("system")
      | first = get_param(sys,'Created');
      | first = first(end-3:end);  %year is last four digits
      | 
      | last = get_param(sys,'LastModifiedDate');
      | if isempty(last)
      |     last = datestr(now,'yyyy');
      | else
      |     last = last(end-3:end);
      | end
      | 
      | if strcmp(first,last)
      |     fprintf('%s -- Copyright %s Nexteer',NxtrConf,first)
      | else
      |     fprintf('%s -- %s%s- %s Nexteer',NxtrConf,char(169),first,last)
      | end
  LimStat_f2 : NxtrLim/LimStat_f32  LoLim=single(0)  HiLim=FILOUTPLIM_ULS_F32
      settings: AttributesFormatString=Lower Limit: %<LoLim>\nUpper Limit: %<HiLim>
  DutyCycleLevel : Outport
  wires:
  LimStat_f2/1 -> DutyCycleLevel/1
  MaxSlowFilt/1 -> LimStat_f2/1

== system SF009A_DutyCycThermProtn/DutyCycThermProtn/DutyCycThermProtnPer1/LoadLimiting/Multiplier/CopyRight2 ==
